simulink model "ADHW8p1"  (R2022b)
settings: Solver=VariableStepAuto  StartTime=0.0  StopTime=5337.0  RelTol=1e-3
settings Model: Creator=izacu  LastModifiedBy=izacu

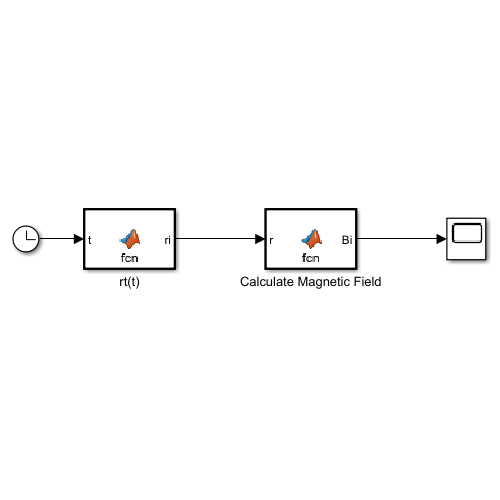
[thumbnail: Simulink's stored preview of the top-level diagram]
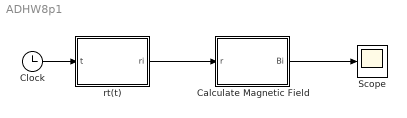
== system ADHW8p1 ==
  Calculate Magnetic Field : MATLAB Function  TreatAsAtomicUnit=on
  Clock : Clock
  Scope : Scope
  rt(t) : MATLAB Function  TreatAsAtomicUnit=on
  wires:
  Clock/1 -> rt(t)/1(t)
  rt(t)/1(ri) -> Calculate Magnetic Field/1(r)
  Calculate Magnetic Field/1(Bi) -> Scope/1

== matlab function ADHW8p1/rt(t) ==
  data: t input; ri output
function ri = fcn(t)

p = 6600;
mu = 398600;
w = sqrt(mu / (p^3));

ri = (p/sqrt(2)) * [-cos(w*t); sqrt(2)*sin(w*t); cos(w*t)];

== matlab function ADHW8p1/Calculate Magnetic Field ==
  data: r input; Bi output
function Bi = fcn(r)

Re = 6378; % km
B0 = 3.12e-5; % T

nz = -r./norm(r);
ny = cross(nz, [0; 0; 1]) ./ norm(cross(nz, [0; 0; 1]));
nx = cross(ny,nz);
Ti2n = [nx'; ny'; nz'];

lat = acos(r(3)/norm(r));

Bn = (B0*(Re/norm(r))^3) * [cos(lat); 0; -2*sin(lat)];

Bi = Ti2n*Bn;
